simulink model "simulation"  (R2017b)
settings: Solver=FixedStepAuto  StartTime=0.0  StopTime=simTotalTime  FixedStep=0.05  MaxStep=0.1  MinStep=0.01  RelTol=1e-3
undefined symbols (not defined in the file): gridArea, gridDen, gridLength, hysteronMax, hysteronMin, initialInput, initialRelays, inputFactor, inputMax, inputMin, offset, outputFactor, outputMax, outputMin, simTotalTime, weightFunc, xyGrid
libraries: simulink x1
settings Model: Creator=Marco  LastModifiedBy=M. Vasquez Beltran

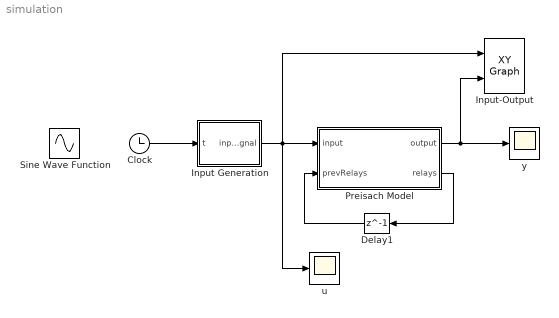
== system simulation ==
  Clock : Clock
  Delay1 : Delay  DelayLength=1  InitialCondition=initialRelays
  Input Generation : MATLAB Function  TreatAsAtomicUnit=on
  Input-Output : simulink/Sinks/XY Graph  xmin=inputMin*inputFactor  xmax=inputMax*inputFactor  ymin=outputMin*outputFactor  ymax=outputMax*outputFactor  st=-1
  Preisach Model : MATLAB Function  TreatAsAtomicUnit=on
  Sine Wave Function : Sin  Amplitude=(inputMax-inputMin)/2  Bias=(inputMax+inputMin)/2  Frequency=3*(2*pi/simTotalTime)  SampleTime=0
  u : Scope
  y : Scope
  wires:
  Preisach Model/1(output) -> Input-Output/2, y/1
  Preisach Model/2(relays) -> Delay1/1
  Delay1/1 -> Preisach Model/2(prevRelays)
  Clock/1 -> Input Generation/1(t)
  Input Generation/1(inputSignal) -> Input-Output/1, u/1, Preisach Model/1(input)

== matlab function simulation/Input Generation ==
  data: t input; inputMin parameter; inputMax parameter; initialInput parameter; simTotalTime parameter; inputSignal output
function inputSignal = fcn(t,...
    inputMin, inputMax, initialInput, simTotalTime)

inputMinFac = 1.00;
inputMaxFac = 1.00;

%Constant amplitude
% amp = 0.25*(inputMaxFac*inputMax - inputMinFac*inputMin)/2; 

%Decreasing amplitude
timeDecFac = ( simTotalTime - 0.75*t )/simTotalTime;
amp = timeDecFac*(inputMaxFac*inputMax - inputMinFac*inputMin)/2;

%Signal params
freq = 10*(2*pi/simTotalTime);
offset = (inputMaxFac*inputMax + inputMinFac*inputMin)/2;
phase = -asin((initialInput - offset)/amp); % Neccesary phasefor initial input
phase = 0;

inputSignal = amp * sin( freq*t - phase ) + offset;

== matlab function simulation/Preisach Model ==
  data: input input; prevRelays input; output output; weightFunc parameter; relays output; offset parameter; hysteronMin parameter; hysteronMax parameter; gridDen parameter; xyGrid parameter; gridLength parameter; gridArea parameter
function [output, relays] = fcn(input, prevRelays, ...
    weightFunc, offset, hysteronMin, hysteronMax, gridDen, xyGrid, gridLength, gridArea)

    relays = prevRelays;
    if( xyGrid(end) <= input )
        relays(:,:) = hysteronMax*fliplr(triu(ones(gridDen, gridDen)));
    elseif( input < xyGrid(1) )
        relays(:,:) = hysteronMin*fliplr(triu(ones(gridDen, gridDen)));
    else
        idx0 = 1;
        while( idx0 <= gridDen-1 )
            if( xyGrid(idx0) <= input && input < xyGrid(idx0+1) )
                col = idx0;
                row = gridDen-idx0+1;

                relays(row:end, 1:col) = hysteronMax*fliplr(triu(ones(col, col)));
                relays(1:row-1, col+1:end) = hysteronMin*fliplr(triu(ones(row-1, row-1)));
                break;
            end
            idx0 = idx0 + 1;
        end
    end
    output = sum(sum(relays(:,:).*weightFunc(:,:)))*gridArea + offset;
    
end
